simulink model "ENGN3223_final_system"  (R2025b)
settings: Solver=VariableStepAuto  StartTime=0.0  StopTime=80.0  RelTol=1e-3
values from neighbouring files (symbols this model uses):
  A = [-2.02     1       0 ... (first row only)    [ENGN3223_code 1.m]    (also in ENGN3223_final.m = [X_u              X_w            0              -g; ENGN3223_updated.m = [X_u              X_w            0              -g)
  B = [0.16 ... (first row only)    [ENGN3223_code 1.m]    (also in ENGN3223_final.m = -[X_del               X_del_T; ENGN3223_updated.m = -[X_del               X_del_T)
  C = [0 0 1]    [ENGN3223_code 1.m]    (also in ENGN3223_final.m = eye(4); ENGN3223_updated.m = eye(4))
  D = 0    [ENGN3223_code 1.m]    (also in ENGN3223_final.m = zeros(4, 2); ENGN3223_updated.m = zeros(4, 2))
  K = acker(A,B,desired_poles)    [ENGN3223_code 1.m]    (also in ENGN3223_final.m = place(A,B,desired_poles); ENGN3223_updated.m = place(A,B,desired_poles))
  N_bar = (1-steady_state_error/100)/G0    [ENGN3223_final.m]
  target_pitch_rad = 10*pi/180    (= 0.174532925199)    [ENGN3223_final.m]    (also in ENGN3223_updated.m = 0.3)

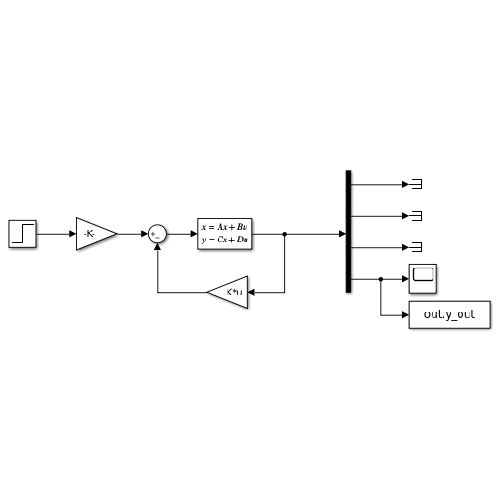
[thumbnail: Simulink's stored preview of the top-level diagram]
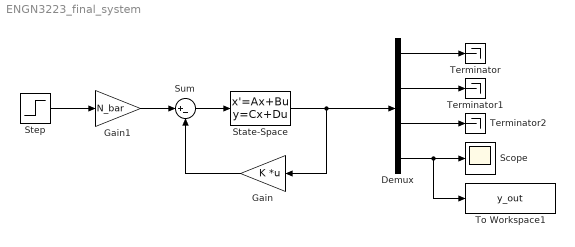
== system ENGN3223_final_system ==
  Demux : Demux
  Gain : Gain  Gain=K  Multiplication=Matrix(K*u)
  Gain1 : Gain  Gain=N_bar
  Scope : Scope
      settings: ActiveDisplayYMinimum=-0.039701490896232178  ActiveDisplayYMaximum=0.35731341806608968
  State-Space : StateSpace  A=A  B=B  C=C  D=D  InitialCondition=0  ContinuousStateAttributes={'Horizontal_velocity','Vertical_velocity','Pitch_rate','Pitch_angle'}
  Step : Step  Time=0  After=target_pitch_rad  SampleTime=0
  Sum : Sum  Inputs=|+-
  Terminator : Terminator
  Terminator1 : Terminator
  Terminator2 : Terminator
  To Workspace1 : ToWorkspace  VariableName=y_out  SaveFormat=Timeseries  SampleTime=-1
  wires:
  Gain/1 -> Sum/2
  Sum/1 -> State-Space/1
  Demux/4 -> Scope/1, To Workspace1/1
  Demux/3 -> Terminator2/1
  State-Space/1 -> Demux/1, Gain/1
  Demux/1 -> Terminator/1
  Demux/2 -> Terminator1/1
  Step/1 -> Gain1/1
  Gain1/1 -> Sum/1
